simulink model "pHRIControl"  (Simulink 8.7)
settings: Solver=ode5  StartTime=0.0  StopTime=inf  FixedStep=0.01  RelTol=1e-3
InitFcn:
  | initpHRIControl
undefined symbols (not defined in the file or in its folder): CONFIG, HUMAN, ROBOT
libraries: WBToolboxLibrary x37
settings Model: Creator=yeshi  LastModifiedBy=yeshi  NumberOfSteps=50
settings DataIOCC: LimitDataPoints=off  SaveFormat=Dataset
settings DebuggingCC: UnderspecifiedInitializationDetection=Simplified  MergeDetectMultiDrivingBlocksExec=error
settings HardwareCC: ProdBitPerPointer=64  ProdLargestAtomicFloat=Float  ProdIntDivRoundTo=Zero  ProdEndianess=LittleEndian  ProdWordSize=64  ProdHWDeviceType=Intel->x86-64 (Windows64)
settings ModelReferenceCC: PropagateSignalLabelsOutOfModel=on
settings ConfigComp: CovModelRefEnable=off

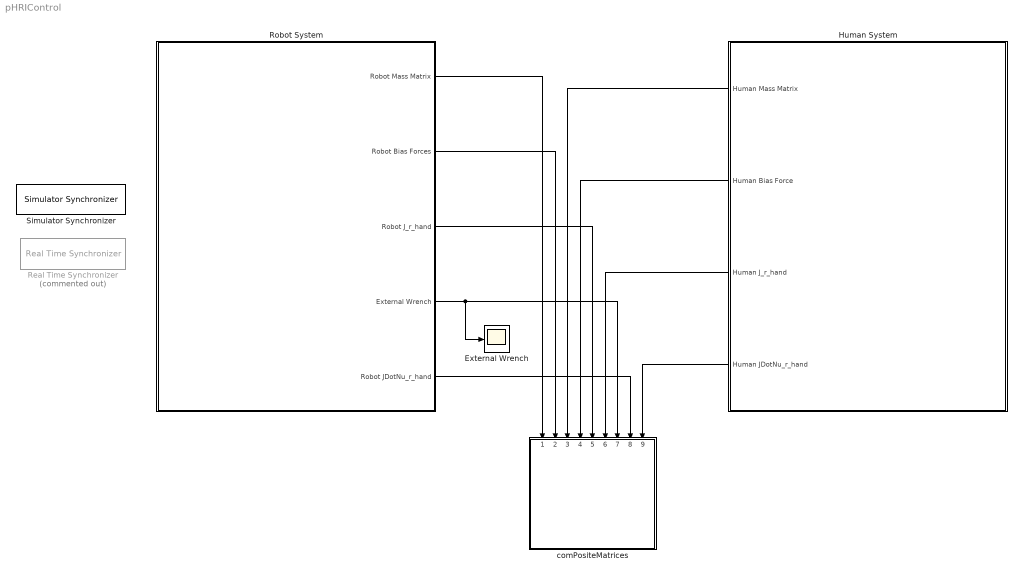
== system pHRIControl ==
  External Wrench : Scope
  Human System : Subsystem
  Real Time Synchronizer : WBToolboxLibrary/Utilities/Real Time Synchronizer  Commented=on  period=0.01
  Robot System : Subsystem
  Simulator Synchronizer : WBToolboxLibrary/Utilities/Simulator Synchronizer  period=0.01  serverPortName='/clock/rpc'  clientPortName='/WBT_synchronizer/rpc:o'
  comPositeMatrices : MATLAB Function  TreatAsAtomicUnit=on
  wires:
  Robot System/2(Robot Bias Forces) -> comPositeMatrices/2(robotBiasForce)
  Robot System/1(Robot Mass Matrix) -> comPositeMatrices/1(robotM)
  Human System/1(Human Mass Matrix) -> comPositeMatrices/3(humanM)
  Human System/2(Human Bias Force) -> comPositeMatrices/4(humanBiasForce)
  Robot System/3(Robot J_r_hand) -> comPositeMatrices/5(robotEEJ)
  Human System/3(Human J_r_hand) -> comPositeMatrices/6(humanEEJ)
  Robot System/5(Robot JDotNu_r_hand) -> comPositeMatrices/8(robotJDotNu)
  Human System/4(Human JDotNu_r_hand) -> comPositeMatrices/9(humanJDotNu)
  Robot System/4(External Wrench) -> External Wrench/1, comPositeMatrices/7(extWrench)

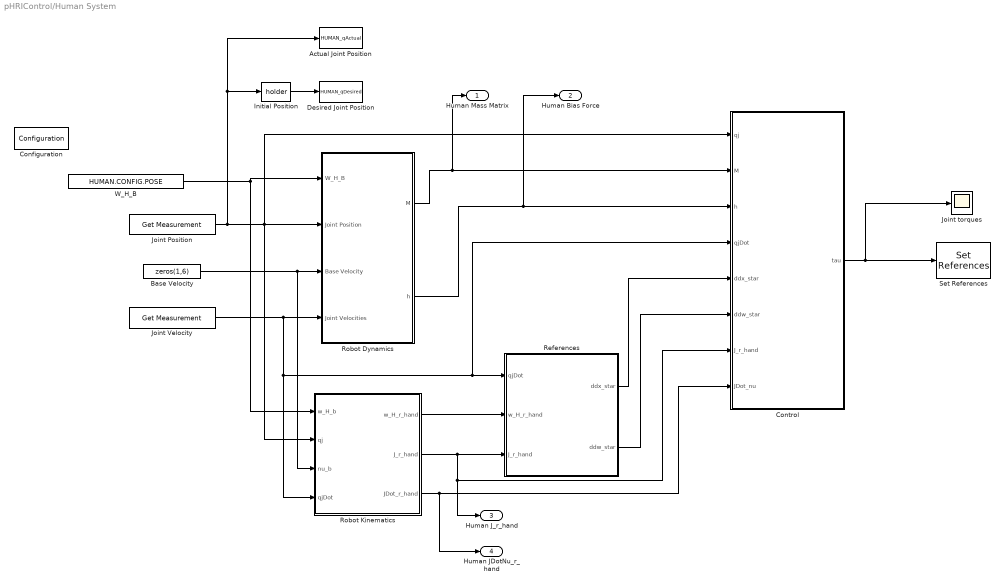
== system pHRIControl/Human System ==
  Actual Joint Position : ToWorkspace  VariableName=HUMAN_qActual  SaveFormat=Timeseries  SampleTime=-1
  "Base Velocity " : Constant  Value=zeros(1,6)
  Configuration : WBToolboxLibrary/Utilities/Configuration  ConfigSource=Workspace  ConfigObject='HUMAN.WBTConfigRobot'
  Control : Subsystem
  Desired Joint Position : ToWorkspace  VariableName=HUMAN_qDesired  SaveFormat=Timeseries  SampleTime=-1
  "Initial Position " : WBToolboxLibrary/Utilities/holder 
  Joint Position : WBToolboxLibrary/wholeBodyStates/Get Measurement  measuredType=Joints Position
  Joint Velocity : WBToolboxLibrary/wholeBodyStates/Get Measurement  measuredType=Joints Velocity
  Joint torques : Scope
  References : Subsystem
  Robot Dynamics : Subsystem
  Robot Kinematics : Subsystem
  Set References : WBToolboxLibrary/wholeBodyActuators/Set References  controlType=Torque  refSpeed=50
  "W_H_B " : Constant  Value=HUMAN.CONFIG.POSE
  Human Mass Matrix : Outport
  Human Bias Force : Outport  Port=2
  Human J_r_hand : Outport  Port=3
  Human JDotNu_r_hand : Outport  Port=4
  wires:
  Robot Dynamics/2(h) -> Human Bias Force/1, Control/3(h)
  "Base Velocity "/1 -> Robot Dynamics/3(Base Velocity), Robot Kinematics/3(nu_b)
  Robot Kinematics/2(J_r_hand) -> Human J_r_hand/1, Control/7(J_r_hand), References/3(J_r_hand)
  "Initial Position "/1 -> Desired Joint Position/1
  References/2(ddw_star) -> Control/6(ddw_star)
  References/1(ddx_star) -> Control/5(ddx_star)
  Control/1(tau) -> Joint torques/1, Set References/1
  Robot Kinematics/3(JDot_r_hand) -> Human JDotNu_r_hand/1, Control/8(JDot_nu)
  Robot Kinematics/1(w_H_r_hand) -> References/2(w_H_r_hand)
  Robot Dynamics/1(M) -> Human Mass Matrix/1, Control/2(M)
  "W_H_B "/1 -> Robot Dynamics/1(W_H_B), Robot Kinematics/1(w_H_b)
  Joint Velocity/1 -> Robot Dynamics/4(" Joint Velocities "), References/1(qjDot), Control/4(qjDot), Robot Kinematics/4(qjDot)
  Joint Position/1 -> "Initial Position "/1, Actual Joint Position/1, Robot Dynamics/2(Joint Position), Control/1(qj), Robot Kinematics/2(qj)

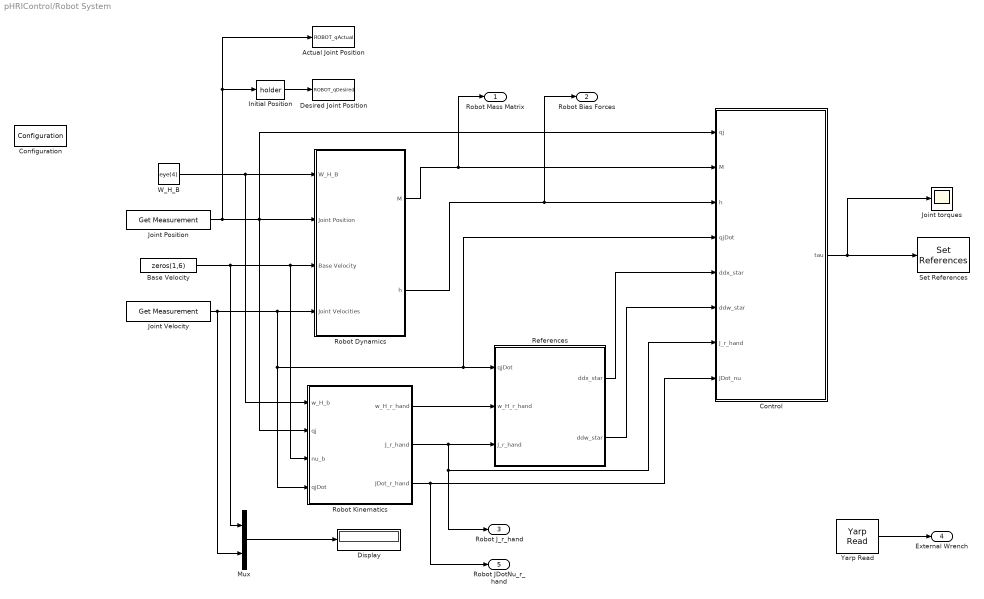
== system pHRIControl/Robot System ==
  Actual Joint Position : ToWorkspace  VariableName=ROBOT_qActual  SaveFormat=Timeseries  SampleTime=-1
  "Base Velocity " : Constant  Value=zeros(1,6)
  Configuration : WBToolboxLibrary/Utilities/Configuration  ConfigSource=Workspace  ConfigObject='ROBOT.WBTConfigRobot'
  Control : Subsystem
  Desired Joint Position : ToWorkspace  VariableName=ROBOT_qDesired  SaveFormat=Timeseries  SampleTime=-1
  Display : Display
  "Initial Position " : WBToolboxLibrary/Utilities/holder 
  Joint Position : WBToolboxLibrary/wholeBodyStates/Get Measurement  measuredType=Joints Position
  Joint Velocity : WBToolboxLibrary/wholeBodyStates/Get Measurement  measuredType=Joints Velocity
  Joint torques : Scope
  Mux : Mux  Inputs=2
  References : Subsystem
  Robot Dynamics : Subsystem
  Robot Kinematics : Subsystem
  Set References : WBToolboxLibrary/wholeBodyActuators/Set References  controlType=Torque  refSpeed=50
  "W_H_B " : Constant  Value=eye(4)
  Yarp Read : WBToolboxLibrary/Utilities/Yarp Read  portName='/iCub/wholeBodyDynamics/right_arm/endEffectorWrench:o'  signalSize=6  blocking=off  timestamp=off  autoconnect=on  errorOnConnection=on
  Robot Mass Matrix : Outport
  Robot Bias Forces : Outport  Port=2
  Robot J_r_hand : Outport  Port=3
  External Wrench : Outport  Port=4
  Robot JDotNu_r_hand : Outport  Port=5
  wires:
  Joint Position/1 -> Robot Kinematics/2(qj), Control/1(qj), Robot Dynamics/2(Joint Position), Actual Joint Position/1, "Initial Position "/1
  Joint Velocity/1 -> Mux/2, Robot Kinematics/4(qjDot), Control/4(qjDot), References/1(qjDot), Robot Dynamics/4(" Joint Velocities ")
  "W_H_B "/1 -> Robot Kinematics/1(w_H_b), Robot Dynamics/1(W_H_B)
  Robot Dynamics/1(M) -> Control/2(M), Robot Mass Matrix/1
  Robot Kinematics/1(w_H_r_hand) -> References/2(w_H_r_hand)
  Robot Kinematics/3(JDot_r_hand) -> Robot JDotNu_r_hand/1, Control/8(JDot_nu)
  Control/1(tau) -> Set References/1, Joint torques/1
  References/1(ddx_star) -> Control/5(ddx_star)
  References/2(ddw_star) -> Control/6(ddw_star)
  "Initial Position "/1 -> Desired Joint Position/1
  Robot Kinematics/2(J_r_hand) -> References/3(J_r_hand), Robot J_r_hand/1, Control/7(J_r_hand)
  "Base Velocity "/1 -> Mux/1, Robot Kinematics/3(nu_b), Robot Dynamics/3(Base Velocity)
  Robot Dynamics/2(h) -> Robot Bias Forces/1, Control/3(h)
  Yarp Read/1 -> External Wrench/1
  Mux/1 -> Display/1

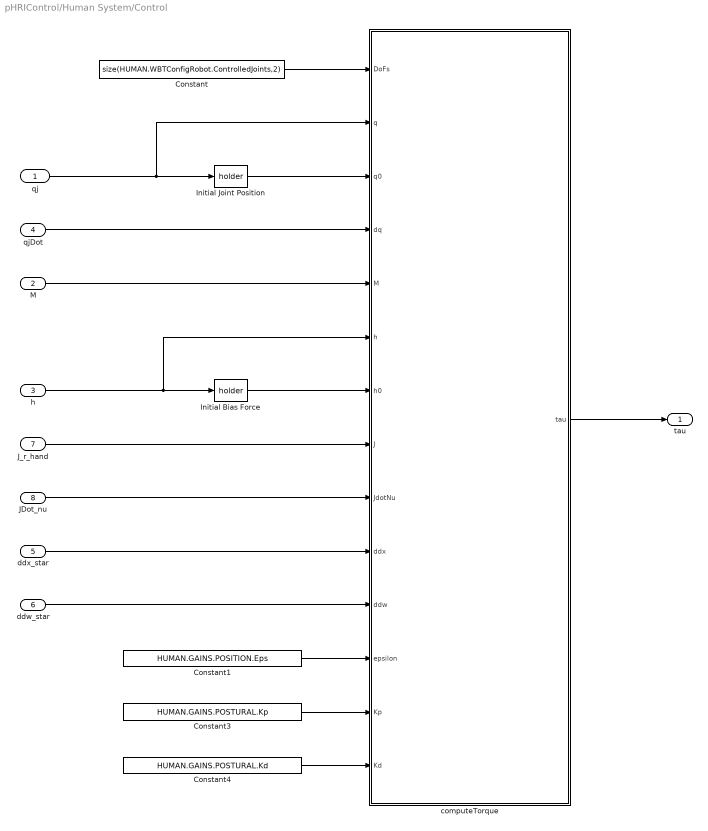
== system pHRIControl/Human System/Control ==
  qj : Inport
  M : Inport  Port=2
  h : Inport  Port=3
  qjDot : Inport  Port=4
  ddx_star : Inport  Port=5
  ddw_star : Inport  Port=6
  J_r_hand : Inport  Port=7
  JDot_nu : Inport  Port=8
  Constant : Constant  Value=size(HUMAN.WBTConfigRobot.ControlledJoints,2)
  Constant1 : Constant  Value=HUMAN.GAINS.POSITION.Eps
  Constant3 : Constant  Value=HUMAN.GAINS.POSTURAL.Kp
  Constant4 : Constant  Value=HUMAN.GAINS.POSTURAL.Kd
  Initial Bias Force : WBToolboxLibrary/Utilities/holder 
  Initial Joint Position : WBToolboxLibrary/Utilities/holder 
  computeTorque : MATLAB Function  TreatAsAtomicUnit=on
  tau : Outport
  wires:
  Constant4/1 -> computeTorque/14(Kd)
  Constant3/1 -> computeTorque/13(Kp)
  Constant1/1 -> computeTorque/12(epsilon)
  ddw_star/1 -> computeTorque/11(ddw)
  M/1 -> computeTorque/5(M)
  J_r_hand/1 -> computeTorque/8(J)
  Initial Joint Position/1 -> computeTorque/3(q0)
  Initial Bias Force/1 -> computeTorque/7(h0)
  h/1 -> Initial Bias Force/1, computeTorque/6(h)
  computeTorque/1(tau) -> tau/1
  Constant/1 -> computeTorque/1(DoFs)
  JDot_nu/1 -> computeTorque/9(JdotNu)
  qjDot/1 -> computeTorque/4(dq)
  qj/1 -> Initial Joint Position/1, computeTorque/2(q)
  ddx_star/1 -> computeTorque/10(ddx)

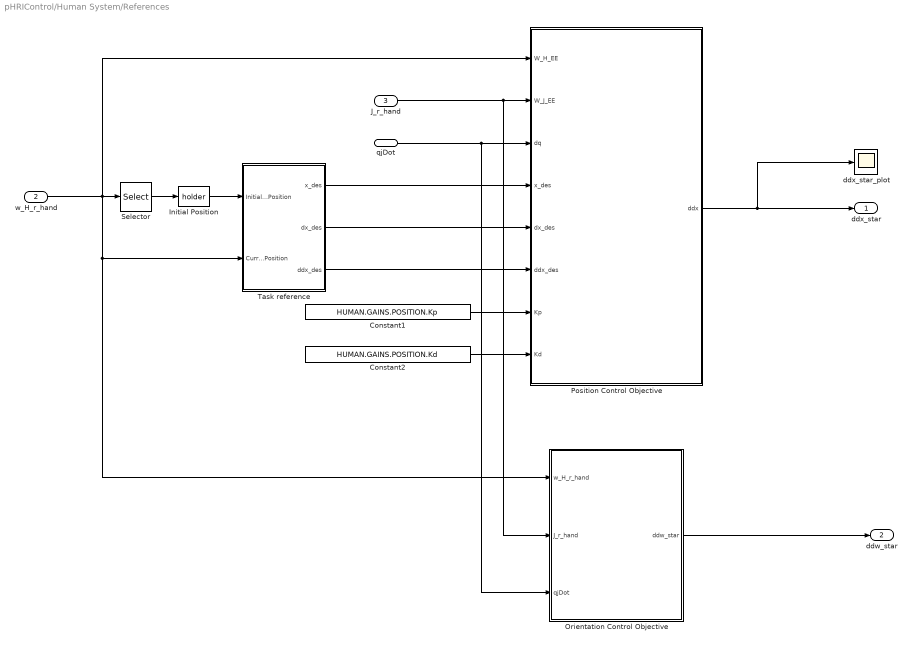
== system pHRIControl/Human System/References ==
  qjDot : Inport
  w_H_r_hand : Inport  Port=2
  J_r_hand : Inport  Port=3
  Constant1 : Constant  Value=HUMAN.GAINS.POSITION.Kp
  Constant2 : Constant  Value=HUMAN.GAINS.POSITION.Kd
  "Initial Position " : WBToolboxLibrary/Utilities/holder 
  Orientation Control Objective : Subsystem
  Position Control Objective : MATLAB Function  TreatAsAtomicUnit=on
  Selector : Selector  NumberOfDimensions=2  InputPortWidth=3  IndexOptions=Index vector (dialog),Index vector (dialog)  Indices=[1 2 3],4  OutputSizes=1,1
  Task reference : Subsystem
  ddx_star_plot : Scope
  ddx_star : Outport
  ddw_star : Outport  Port=2
  wires:
  Orientation Control Objective/1(ddw_star) -> ddw_star/1
  Constant2/1 -> Position Control Objective/8(Kd)
  Constant1/1 -> Position Control Objective/7(Kp)
  w_H_r_hand/1 -> Task reference/2(Current Position), Orientation Control Objective/1(w_H_r_hand), Position Control Objective/1(W_H_EE), Selector/1
  qjDot/1 -> Position Control Objective/3(dq), Orientation Control Objective/3(qjDot)
  Selector/1 -> "Initial Position "/1
  Position Control Objective/1(ddx) -> ddx_star_plot/1, ddx_star/1
  "Initial Position "/1 -> Task reference/1(Initial Position)
  Task reference/3(ddx_des) -> Position Control Objective/6(ddx_des)
  Task reference/2(dx_des) -> Position Control Objective/5(dx_des)
  Task reference/1(x_des) -> Position Control Objective/4(x_des)
  J_r_hand/1 -> Position Control Objective/2(W_J_EE), Orientation Control Objective/2(J_r_hand)

== system pHRIControl/Human System/Robot Dynamics ==
  W_H_B : Inport
  Joint Position : Inport  Port=2
  Base Velocity : Inport  Port=3
  " Joint Velocities " : Inport  Port=4
  Get Bias Forces : WBToolboxLibrary/wholeBodyModel/Dynamics/Get Bias Forces
  Mass Matrix : WBToolboxLibrary/wholeBodyModel/Dynamics/Mass Matrix
  M : Outport
  h : Outport  Port=2
  wires:
  Mass Matrix/1 -> M/1
  Base Velocity/1 -> Get Bias Forces/3
  W_H_B/1 -> Get Bias Forces/1, Mass Matrix/1
  Get Bias Forces/1 -> h/1
  " Joint Velocities "/1 -> Get Bias Forces/4
  Joint Position/1 -> Get Bias Forces/2, Mass Matrix/2

== system pHRIControl/Human System/Robot Kinematics ==
  w_H_b : Inport
  qj : Inport  Port=2
  nu_b : Inport  Port=3
  qjDot : Inport  Port=4
  DotJ Nu : WBToolboxLibrary/wholeBodyModel/Jacobians/DotJ Nu  frameName=HUMAN.CONFIG.EE
  Forward Kinematics : WBToolboxLibrary/wholeBodyModel/Kinematics/Forward Kinematics  frameName=HUMAN.CONFIG.EE
  Jacobian 6x(6+n) : WBToolboxLibrary/wholeBodyModel/Jacobians/Jacobian  frameName=HUMAN.CONFIG.EE
  w_H_r_hand : Outport
  J_r_hand : Outport  Port=2
  JDot_r_hand : Outport  Port=3
  wires:
  DotJ Nu/1 -> JDot_r_hand/1
  Forward Kinematics/1 -> w_H_r_hand/1
  Jacobian 6x(6+n)/1 -> J_r_hand/1
  nu_b/1 -> DotJ Nu/3
  qjDot/1 -> DotJ Nu/4
  qj/1 -> Forward Kinematics/2, Jacobian 6x(6+n)/2, DotJ Nu/2
  w_H_b/1 -> Forward Kinematics/1, Jacobian 6x(6+n)/1, DotJ Nu/1

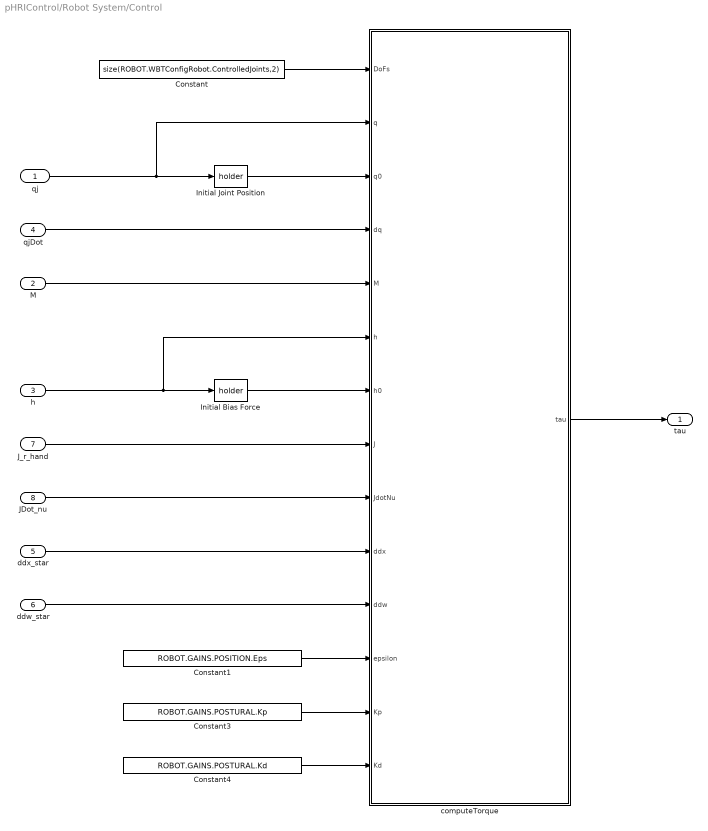
== system pHRIControl/Robot System/Control ==
  qj : Inport
  M : Inport  Port=2
  h : Inport  Port=3
  qjDot : Inport  Port=4
  ddx_star : Inport  Port=5
  ddw_star : Inport  Port=6
  J_r_hand : Inport  Port=7
  JDot_nu : Inport  Port=8
  Constant : Constant  Value=size(ROBOT.WBTConfigRobot.ControlledJoints,2)
  Constant1 : Constant  Value=ROBOT.GAINS.POSITION.Eps
  Constant3 : Constant  Value=ROBOT.GAINS.POSTURAL.Kp
  Constant4 : Constant  Value=ROBOT.GAINS.POSTURAL.Kd
  Initial Bias Force : WBToolboxLibrary/Utilities/holder 
  Initial Joint Position : WBToolboxLibrary/Utilities/holder 
  computeTorque : MATLAB Function  TreatAsAtomicUnit=on
  tau : Outport
  wires:
  ddx_star/1 -> computeTorque/10(ddx)
  qj/1 -> computeTorque/2(q), Initial Joint Position/1
  qjDot/1 -> computeTorque/4(dq)
  JDot_nu/1 -> computeTorque/9(JdotNu)
  Constant/1 -> computeTorque/1(DoFs)
  computeTorque/1(tau) -> tau/1
  h/1 -> computeTorque/6(h), Initial Bias Force/1
  Initial Bias Force/1 -> computeTorque/7(h0)
  Initial Joint Position/1 -> computeTorque/3(q0)
  J_r_hand/1 -> computeTorque/8(J)
  M/1 -> computeTorque/5(M)
  ddw_star/1 -> computeTorque/11(ddw)
  Constant1/1 -> computeTorque/12(epsilon)
  Constant3/1 -> computeTorque/13(Kp)
  Constant4/1 -> computeTorque/14(Kd)

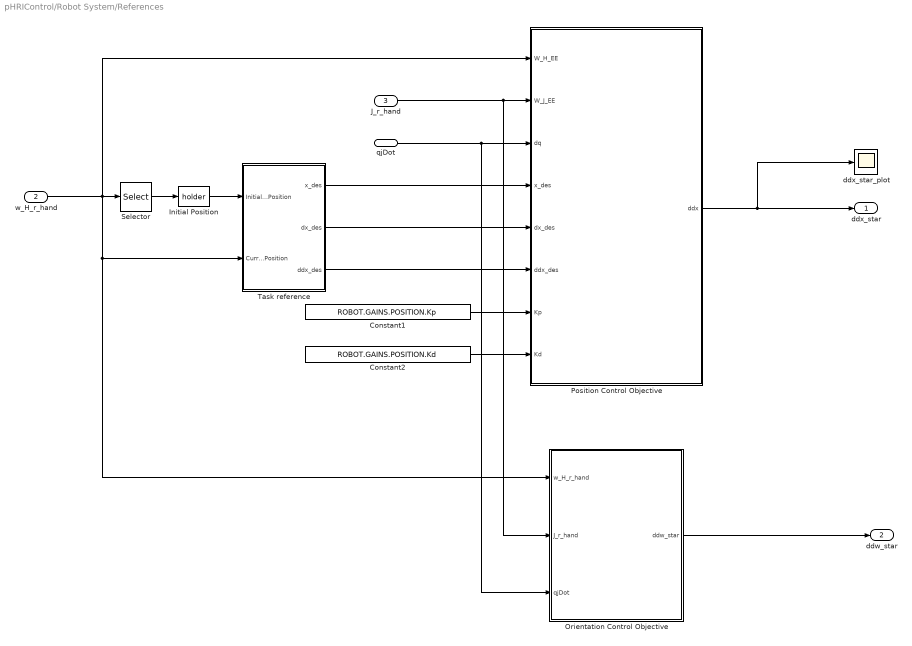
== system pHRIControl/Robot System/References ==
  qjDot : Inport
  w_H_r_hand : Inport  Port=2
  J_r_hand : Inport  Port=3
  Constant1 : Constant  Value=ROBOT.GAINS.POSITION.Kp
  Constant2 : Constant  Value=ROBOT.GAINS.POSITION.Kd
  "Initial Position " : WBToolboxLibrary/Utilities/holder 
  Orientation Control Objective : Subsystem
  Position Control Objective : MATLAB Function  TreatAsAtomicUnit=on
  Selector : Selector  NumberOfDimensions=2  InputPortWidth=3  IndexOptions=Index vector (dialog),Index vector (dialog)  Indices=[1 2 3],4  OutputSizes=1,1
  Task reference : Subsystem
  ddx_star_plot : Scope
  ddx_star : Outport
  ddw_star : Outport  Port=2
  wires:
  J_r_hand/1 -> Orientation Control Objective/2(J_r_hand), Position Control Objective/2(W_J_EE)
  Task reference/1(x_des) -> Position Control Objective/4(x_des)
  Task reference/2(dx_des) -> Position Control Objective/5(dx_des)
  Task reference/3(ddx_des) -> Position Control Objective/6(ddx_des)
  "Initial Position "/1 -> Task reference/1(Initial Position)
  Position Control Objective/1(ddx) -> ddx_star/1, ddx_star_plot/1
  Selector/1 -> "Initial Position "/1
  qjDot/1 -> Orientation Control Objective/3(qjDot), Position Control Objective/3(dq)
  w_H_r_hand/1 -> Selector/1, Position Control Objective/1(W_H_EE), Orientation Control Objective/1(w_H_r_hand), Task reference/2(Current Position)
  Constant1/1 -> Position Control Objective/7(Kp)
  Constant2/1 -> Position Control Objective/8(Kd)
  Orientation Control Objective/1(ddw_star) -> ddw_star/1

== system pHRIControl/Robot System/Robot Dynamics ==
  W_H_B : Inport
  Joint Position : Inport  Port=2
  Base Velocity : Inport  Port=3
  " Joint Velocities " : Inport  Port=4
  Get Bias Forces : WBToolboxLibrary/wholeBodyModel/Dynamics/Get Bias Forces
  Mass Matrix : WBToolboxLibrary/wholeBodyModel/Dynamics/Mass Matrix
  M : Outport
  h : Outport  Port=2
  wires:
  Joint Position/1 -> Mass Matrix/2, Get Bias Forces/2
  " Joint Velocities "/1 -> Get Bias Forces/4
  Get Bias Forces/1 -> h/1
  W_H_B/1 -> Mass Matrix/1, Get Bias Forces/1
  Base Velocity/1 -> Get Bias Forces/3
  Mass Matrix/1 -> M/1

== system pHRIControl/Robot System/Robot Kinematics ==
  w_H_b : Inport
  qj : Inport  Port=2
  nu_b : Inport  Port=3
  qjDot : Inport  Port=4
  DotJ Nu : WBToolboxLibrary/wholeBodyModel/Jacobians/DotJ Nu  frameName=ROBOT.CONFIG.EE
  Forward Kinematics : WBToolboxLibrary/wholeBodyModel/Kinematics/Forward Kinematics  frameName=ROBOT.CONFIG.EE
  Jacobian 6x(6+n) : WBToolboxLibrary/wholeBodyModel/Jacobians/Jacobian  frameName=ROBOT.CONFIG.EE
  w_H_r_hand : Outport
  J_r_hand : Outport  Port=2
  JDot_r_hand : Outport  Port=3
  wires:
  w_H_b/1 -> DotJ Nu/1, Jacobian 6x(6+n)/1, Forward Kinematics/1
  qj/1 -> DotJ Nu/2, Jacobian 6x(6+n)/2, Forward Kinematics/2
  qjDot/1 -> DotJ Nu/4
  nu_b/1 -> DotJ Nu/3
  Jacobian 6x(6+n)/1 -> J_r_hand/1
  Forward Kinematics/1 -> w_H_r_hand/1
  DotJ Nu/1 -> JDot_r_hand/1

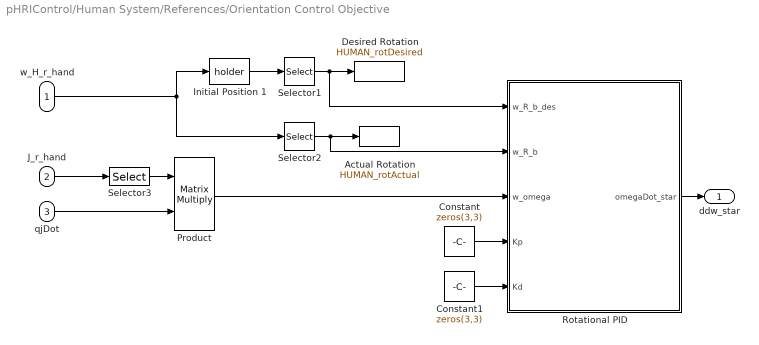
== system pHRIControl/Human System/References/Orientation Control Objective ==
  w_H_r_hand : Inport
  J_r_hand : Inport  Port=2
  qjDot : Inport  Port=3
  Actual Rotation : ToWorkspace  VariableName=HUMAN_rotActual  SaveFormat=Timeseries  SampleTime=-1
  Constant : Constant  Value=zeros(3,3)
  Constant1 : Constant  Value=zeros(3,3)
  Desired Rotation : ToWorkspace  VariableName=HUMAN_rotDesired  SaveFormat=Timeseries  SampleTime=-1
  Initial Position 1 : WBToolboxLibrary/Utilities/holder 
  Product : Product  Multiplication=Matrix(*)
  Rotational PID : MATLAB Function  TreatAsAtomicUnit=on
  Selector1 : Selector  NumberOfDimensions=2  InputPortWidth=4  IndexOptions=Index vector (dialog),Index vector (dialog)  Indices=[1:3],[1:3]  OutputSizes=1,1
  Selector2 : Selector  NumberOfDimensions=2  InputPortWidth=4  IndexOptions=Index vector (dialog),Index vector (dialog)  Indices=[1:3],[1:3]  OutputSizes=1,1
  Selector3 : Selector  NumberOfDimensions=2  InputPortWidth=4  IndexOptions=Index vector (dialog),Index vector (dialog)  Indices=[4:6],[7:6+11]  OutputSizes=1,1
  ddw_star : Outport
  wires:
  Product/1 -> Rotational PID/3(w_omega)
  qjDot/1 -> Product/2
  Selector3/1 -> Product/1
  J_r_hand/1 -> Selector3/1
  Constant1/1 -> Rotational PID/5(Kd)
  Constant/1 -> Rotational PID/4(Kp)
  Initial Position 1/1 -> Selector1/1
  w_H_r_hand/1 -> Initial Position 1/1, Selector2/1
  Selector1/1 -> Rotational PID/1(w_R_b_des), Desired Rotation/1
  Rotational PID/1(omegaDot_star) -> ddw_star/1
  Selector2/1 -> Actual Rotation/1, Rotational PID/2(w_R_b)

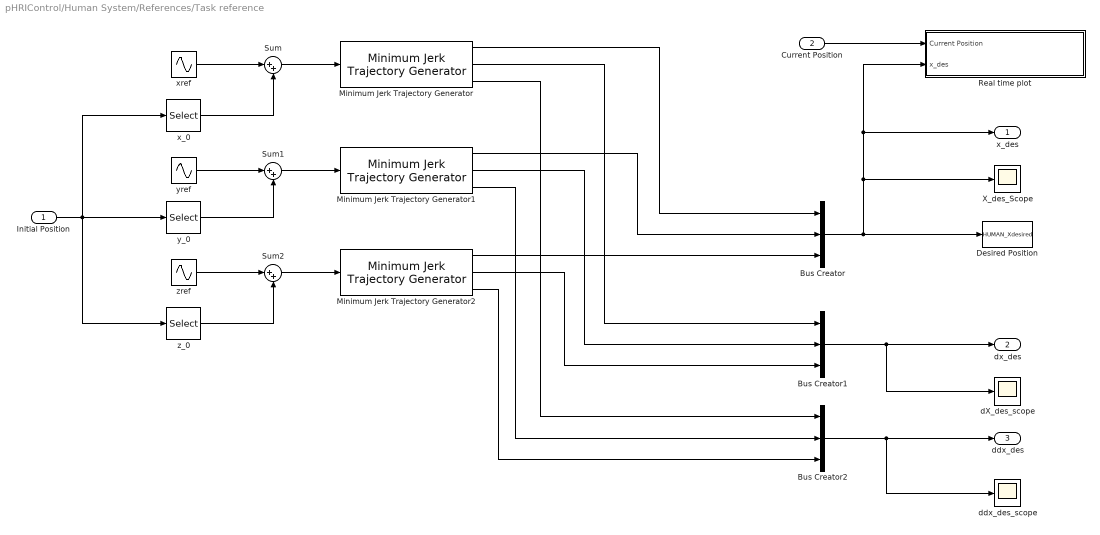
== system pHRIControl/Human System/References/Task reference ==
  Initial Position : Inport
  Current Position : Inport  Port=2
  Bus Creator : BusCreator  Inputs=3
  Bus Creator1 : BusCreator  Inputs=3
  Bus Creator2 : BusCreator  Inputs=3
  Desired Position : ToWorkspace  VariableName=HUMAN_Xdesired  SaveFormat=Timeseries  SampleTime=-1
  Minimum Jerk Trajectory Generator : WBToolboxLibrary/Utilities/Minimum Jerk Trajectory Generator  externalSettlingTime=off  settlingTime=3  sampleTime=0.01  resetOnSettlingTime=off  firstDerivatives=on  secondDerivatives=on  explicitInitialValue=off
  Minimum Jerk Trajectory Generator1 : WBToolboxLibrary/Utilities/Minimum Jerk Trajectory Generator  externalSettlingTime=off  settlingTime=3  sampleTime=0.01  resetOnSettlingTime=off  firstDerivatives=on  secondDerivatives=on  explicitInitialValue=off
  Minimum Jerk Trajectory Generator2 : WBToolboxLibrary/Utilities/Minimum Jerk Trajectory Generator  externalSettlingTime=off  settlingTime=3  sampleTime=0.01  resetOnSettlingTime=off  firstDerivatives=on  secondDerivatives=on  explicitInitialValue=off
  Real time plot : Subsystem
  Sum : Sum  Inputs=|++
  Sum1 : Sum  Inputs=|++
  Sum2 : Sum  Inputs=|++
  X_des_Scope : Scope
  dX_des_scope : Scope
  ddx_des_scope : Scope
  x_0 : Selector  InputPortWidth=3  IndexOptions=Index vector (dialog)  Indices=[1]  OutputSizes=1
  xref : Sin  Amplitude=0  SampleTime=0
  y_0 : Selector  InputPortWidth=3  IndexOptions=Index vector (dialog)  Indices=[2]  OutputSizes=1
  yref : Sin  Amplitude=0  SampleTime=0
  z_0 : Selector  InputPortWidth=3  IndexOptions=Index vector (dialog)  Indices=[3]  OutputSizes=1
  zref : Sin  Amplitude=0  Phase=pi/2  SampleTime=0
  x_des : Outport
  dx_des : Outport  Port=2
  ddx_des : Outport  Port=3
  wires:
  Current Position/1 -> Real time plot/1(Current Position)
  x_0/1 -> Sum/2
  Initial Position/1 -> z_0/1, y_0/1, x_0/1
  z_0/1 -> Sum2/2
  Sum/1 -> Minimum Jerk Trajectory Generator/1
  Minimum Jerk Trajectory Generator/2 -> Bus Creator1/1
  xref/1 -> Sum/1
  Minimum Jerk Trajectory Generator1/1 -> Bus Creator/2
  Bus Creator/1 -> X_des_Scope/1, x_des/1, Real time plot/2(x_des), Desired Position/1
  Bus Creator2/1 -> ddx_des_scope/1, ddx_des/1
  Minimum Jerk Trajectory Generator1/2 -> Bus Creator1/2
  zref/1 -> Sum2/1
  Bus Creator1/1 -> dX_des_scope/1, dx_des/1
  Minimum Jerk Trajectory Generator2/3 -> Bus Creator2/3
  Sum1/1 -> Minimum Jerk Trajectory Generator1/1
  y_0/1 -> Sum1/2
  Minimum Jerk Trajectory Generator1/3 -> Bus Creator2/2
  Minimum Jerk Trajectory Generator/1 -> Bus Creator/1
  yref/1 -> Sum1/1
  Minimum Jerk Trajectory Generator/3 -> Bus Creator2/1
  Minimum Jerk Trajectory Generator2/1 -> Bus Creator/3
  Sum2/1 -> Minimum Jerk Trajectory Generator2/1
  Minimum Jerk Trajectory Generator2/2 -> Bus Creator1/3

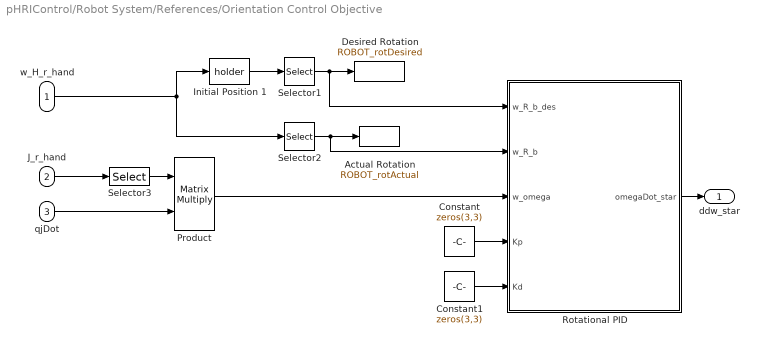
== system pHRIControl/Robot System/References/Orientation Control Objective ==
  w_H_r_hand : Inport
  J_r_hand : Inport  Port=2
  qjDot : Inport  Port=3
  Actual Rotation : ToWorkspace  VariableName=ROBOT_rotActual  SaveFormat=Timeseries  SampleTime=-1
  Constant : Constant  Value=zeros(3,3)
  Constant1 : Constant  Value=zeros(3,3)
  Desired Rotation : ToWorkspace  VariableName=ROBOT_rotDesired  SaveFormat=Timeseries  SampleTime=-1
  Initial Position 1 : WBToolboxLibrary/Utilities/holder 
  Product : Product  Multiplication=Matrix(*)
  Rotational PID : MATLAB Function  TreatAsAtomicUnit=on
  Selector1 : Selector  NumberOfDimensions=2  InputPortWidth=4  IndexOptions=Index vector (dialog),Index vector (dialog)  Indices=[1:3],[1:3]  OutputSizes=1,1
  Selector2 : Selector  NumberOfDimensions=2  InputPortWidth=4  IndexOptions=Index vector (dialog),Index vector (dialog)  Indices=[1:3],[1:3]  OutputSizes=1,1
  Selector3 : Selector  NumberOfDimensions=2  InputPortWidth=4  IndexOptions=Index vector (dialog),Index vector (dialog)  Indices=[4:6],[7:6+11]  OutputSizes=1,1
  ddw_star : Outport
  wires:
  Selector2/1 -> Rotational PID/2(w_R_b), Actual Rotation/1
  Rotational PID/1(omegaDot_star) -> ddw_star/1
  Selector1/1 -> Desired Rotation/1, Rotational PID/1(w_R_b_des)
  w_H_r_hand/1 -> Selector2/1, Initial Position 1/1
  Initial Position 1/1 -> Selector1/1
  Constant/1 -> Rotational PID/4(Kp)
  Constant1/1 -> Rotational PID/5(Kd)
  J_r_hand/1 -> Selector3/1
  Selector3/1 -> Product/1
  qjDot/1 -> Product/2
  Product/1 -> Rotational PID/3(w_omega)

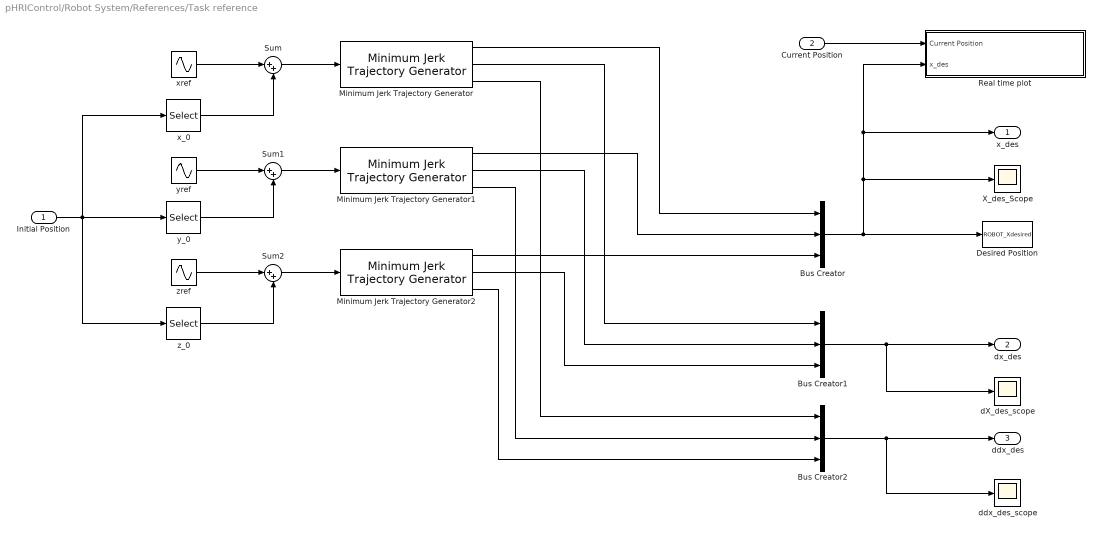
== system pHRIControl/Robot System/References/Task reference ==
  Initial Position : Inport
  Current Position : Inport  Port=2
  Bus Creator : BusCreator  Inputs=3
  Bus Creator1 : BusCreator  Inputs=3
  Bus Creator2 : BusCreator  Inputs=3
  Desired Position : ToWorkspace  VariableName=ROBOT_Xdesired  SaveFormat=Timeseries  SampleTime=-1
  Minimum Jerk Trajectory Generator : WBToolboxLibrary/Utilities/Minimum Jerk Trajectory Generator  externalSettlingTime=off  settlingTime=3  sampleTime=0.01  resetOnSettlingTime=off  firstDerivatives=on  secondDerivatives=on  explicitInitialValue=off
  Minimum Jerk Trajectory Generator1 : WBToolboxLibrary/Utilities/Minimum Jerk Trajectory Generator  externalSettlingTime=off  settlingTime=3  sampleTime=0.01  resetOnSettlingTime=off  firstDerivatives=on  secondDerivatives=on  explicitInitialValue=off
  Minimum Jerk Trajectory Generator2 : WBToolboxLibrary/Utilities/Minimum Jerk Trajectory Generator  externalSettlingTime=off  settlingTime=3  sampleTime=0.01  resetOnSettlingTime=off  firstDerivatives=on  secondDerivatives=on  explicitInitialValue=off
  Real time plot : Subsystem
  Sum : Sum  Inputs=|++
  Sum1 : Sum  Inputs=|++
  Sum2 : Sum  Inputs=|++
  X_des_Scope : Scope
  dX_des_scope : Scope
  ddx_des_scope : Scope
  x_0 : Selector  InputPortWidth=3  IndexOptions=Index vector (dialog)  Indices=[1]  OutputSizes=1
  xref : Sin  Amplitude=0  SampleTime=0
  y_0 : Selector  InputPortWidth=3  IndexOptions=Index vector (dialog)  Indices=[2]  OutputSizes=1
  yref : Sin  Amplitude=0.15  SampleTime=0
  z_0 : Selector  InputPortWidth=3  IndexOptions=Index vector (dialog)  Indices=[3]  OutputSizes=1
  zref : Sin  Amplitude=0  Phase=pi/2  SampleTime=0
  x_des : Outport
  dx_des : Outport  Port=2
  ddx_des : Outport  Port=3
  wires:
  Minimum Jerk Trajectory Generator2/2 -> Bus Creator1/3
  Sum2/1 -> Minimum Jerk Trajectory Generator2/1
  Minimum Jerk Trajectory Generator2/1 -> Bus Creator/3
  Minimum Jerk Trajectory Generator/3 -> Bus Creator2/1
  yref/1 -> Sum1/1
  Minimum Jerk Trajectory Generator/1 -> Bus Creator/1
  Minimum Jerk Trajectory Generator1/3 -> Bus Creator2/2
  y_0/1 -> Sum1/2
  Sum1/1 -> Minimum Jerk Trajectory Generator1/1
  Minimum Jerk Trajectory Generator2/3 -> Bus Creator2/3
  Bus Creator1/1 -> dx_des/1, dX_des_scope/1
  zref/1 -> Sum2/1
  Minimum Jerk Trajectory Generator1/2 -> Bus Creator1/2
  Bus Creator2/1 -> ddx_des/1, ddx_des_scope/1
  Bus Creator/1 -> Desired Position/1, Real time plot/2(x_des), x_des/1, X_des_Scope/1
  Minimum Jerk Trajectory Generator1/1 -> Bus Creator/2
  xref/1 -> Sum/1
  Minimum Jerk Trajectory Generator/2 -> Bus Creator1/1
  Sum/1 -> Minimum Jerk Trajectory Generator/1
  z_0/1 -> Sum2/2
  Initial Position/1 -> x_0/1, y_0/1, z_0/1
  x_0/1 -> Sum/2
  Current Position/1 -> Real time plot/1(Current Position)

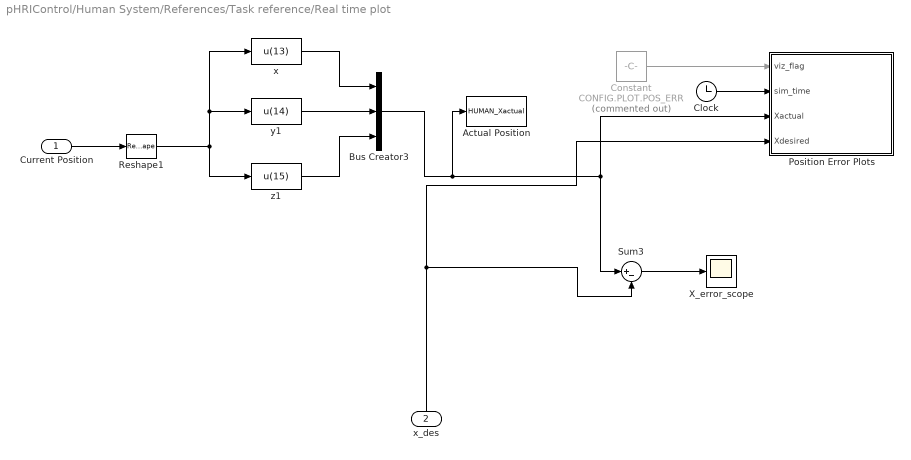
== system pHRIControl/Human System/References/Task reference/Real time plot ==
  Current Position : Inport
  x_des : Inport  Port=2
  Actual Position : ToWorkspace  VariableName=HUMAN_Xactual  SaveFormat=Timeseries  SampleTime=-1
  Bus Creator3 : BusCreator  Inputs=3
  Clock : Clock
  Constant : Constant  Commented=on  Value=CONFIG.PLOT.POS_ERR
  "Position Error Plots " : MATLAB Function  TreatAsAtomicUnit=on
  Reshape1 : Reshape
  Sum3 : Sum  Inputs=|+-
  X_error_scope : Scope
  x : Fcn  Expr=u(13)
  y1 : Fcn  Expr=u(14)
  z1 : Fcn  Expr=u(15)
  wires:
  Sum3/1 -> X_error_scope/1
  Constant/1 -> "Position Error Plots "/1(viz_flag)
  Bus Creator3/1 -> "Position Error Plots "/3(Xactual), Sum3/1, Actual Position/1
  Clock/1 -> "Position Error Plots "/2(sim_time)
  z1/1 -> Bus Creator3/3
  y1/1 -> Bus Creator3/2
  x/1 -> Bus Creator3/1
  Reshape1/1 -> z1/1, y1/1, x/1
  Current Position/1 -> Reshape1/1
  x_des/1 -> "Position Error Plots "/4(Xdesired), Sum3/2

== system pHRIControl/Robot System/References/Task reference/Real time plot ==
  Current Position : Inport
  x_des : Inport  Port=2
  Actual Position : ToWorkspace  VariableName=ROBOT_Xactual  SaveFormat=Timeseries  SampleTime=-1
  Bus Creator3 : BusCreator  Inputs=3
  Clock : Clock
  Constant : Constant  Commented=on  Value=CONFIG.PLOT.POS_ERR
  "Position Error Plots " : MATLAB Function  TreatAsAtomicUnit=on
  Reshape1 : Reshape
  Sum3 : Sum  Inputs=|+-
  X_error_scope : Scope
  x : Fcn  Expr=u(13)
  y1 : Fcn  Expr=u(14)
  z1 : Fcn  Expr=u(15)
  wires:
  x_des/1 -> Sum3/2, "Position Error Plots "/4(Xdesired)
  Current Position/1 -> Reshape1/1
  Reshape1/1 -> x/1, y1/1, z1/1
  x/1 -> Bus Creator3/1
  y1/1 -> Bus Creator3/2
  z1/1 -> Bus Creator3/3
  Clock/1 -> "Position Error Plots "/2(sim_time)
  Bus Creator3/1 -> Actual Position/1, Sum3/1, "Position Error Plots "/3(Xactual)
  Constant/1 -> "Position Error Plots "/1(viz_flag)
  Sum3/1 -> X_error_scope/1

== matlab function Robot System/References/Position Control Objective ==
  data: W_H_EE input double; ddx output double; W_J_EE input double; dq input double; x_des input double; dx_des input double; ddx_des input double; Kp input double; Kd input double
function ddx = controlObjective(W_H_EE,W_J_EE,dq,x_des,dx_des,ddx_des,Kp,Kd)
   
    x  = W_H_EE(1:3,4)-x_des;
    dx = W_J_EE(1:3,7:end)*dq-dx_des;
    
    ddx = ddx_des-Kp*x-Kd*dx; 

end

== matlab function Robot System/Control/computeTorque ==
  data: DoFs input double; q input double; q0 input double; dq input double; M input double; h input double; h0 input double; J input double; JdotNu input double; ddx input double; tau output double; ddw input double; epsilon input double; Kp input double; Kd input double
function tau   = computeTorque(DoFs,q,q0,dq,M,h,h0,J,JdotNu,ddx,ddw,epsilon,Kp,Kd)

    Dofs = 11;
    
    Sb = zeros(Dofs,6);
    Ss = eye(Dofs);
    S = [Sb Ss]';

    ddX = [ddx' 0 0 0]';

    %%Primary Task
    lambda = (J(1:3,:)/M)*S;
    alpha = pinvDamped(lambda,epsilon);
    
    tau_pri = alpha*(ddX(1:3) - JdotNu(1:3) + (J(1:3,:)/M)*h);
    
    nullspace = eye(size(lambda,2)) - alpha*lambda;
    
    %%Postural Task
    kp = Kp;
    kd = Kd;
    tau_null = S'*h - kp*(q-q0) - kd*(dq);
    
    tau = tau_pri + nullspace*tau_null;

end

== matlab function Robot System/References/Task reference/Real time plot/Position Error Plots  ==
  data: viz_flag input double; sim_time input double; Xactual input double; Xdesired input double
function positionErrorPlots(viz_flag,sim_time,Xactual,Xdesired)
%#codegen

coder.extrinsic('animatedline')
coder.extrinsic('addpoints')
coder.extrinsic('legend')
coder.extrinsic('clearpoints')

if(viz_flag ~= 0)
    
    Xerror = Xactual - Xdesired;
    curve_position_error = animatedline('LineWidth',0.1,'Marker','+');

    if(sim_time == 0)
    
        clf;
        close;
    
        fig1 = figure;
        view(177,15); hold on;
        grid on;
        xlabel('x');
        ylabel('y');
        zlabel('z');
        title('Position Error'); hold on;
% %         axis([-0.3 0.3 -0.3 0.3 -0.3 0.3]);
       
    end
    
    figure(1);
    addpoints(curve_position_error,Xerror(1),Xerror(2),Xerror(3));
    drawnow;
    
end

end

== matlab function Robot System/References/Orientation Control Objective/Rotational PID ==
  data: w_R_b_des input double; w_R_b input double; w_omega input double; omegaDot_star output double; Kp input double; Kd input double
function omegaDot_star = rotPID(w_R_b_des,w_R_b,w_omega,Kp,Kd)

    w_omega_des = [0;0;0];
    w_omegaDot_des = [0;0;0];
    
    omegaDot_star = rotationalPID(w_R_b,w_omega,w_R_b_des,w_omega_des,w_omegaDot_des,Kp,Kd);
end

== matlab function Human System/Control/computeTorque ==
  data: DoFs input double; q input double; q0 input double; dq input double; M input double; h input double; h0 input double; J input double; JdotNu input double; ddx input double; tau output double; ddw input double; epsilon input double; Kp input double; Kd input double
function tau   = computeTorque(DoFs,q,q0,dq,M,h,h0,J,JdotNu,ddx,ddw,epsilon,Kp,Kd)

    Dofs = 11;
    
    Sb = zeros(Dofs,6);
    Ss = eye(Dofs);
    S = [Sb Ss]';

    ddX = [ddx' 0 0 0]';

    %%Primary Task
    lambda = (J(1:3,:)/M)*S;
    alpha = pinvDamped(lambda,epsilon);
    
    tau_pri = alpha*(ddX(1:3) - JdotNu(1:3) + (J(1:3,:)/M)*h);
    
    nullspace = eye(size(lambda,2)) - alpha*lambda;
    
    %%Postural Task
    kp = Kp;
    kd = Kd;
    tau_null = S'*h - kp*(q-q0) - kd*(dq);
    
    tau = tau_pri + nullspace*tau_null;

end

== matlab function Human System/References/Orientation Control Objective/Rotational PID ==
  data: w_R_b_des input double; w_R_b input double; w_omega input double; omegaDot_star output double; Kp input double; Kd input double
function omegaDot_star = rotPID(w_R_b_des,w_R_b,w_omega,Kp,Kd)

    w_omega_des = [0;0;0];
    w_omegaDot_des = [0;0;0];
    
    omegaDot_star = rotationalPID(w_R_b,w_omega,w_R_b_des,w_omega_des,w_omegaDot_des,Kp,Kd);
end

== matlab function Human System/References/Position Control Objective ==
  data: W_H_EE input double; ddx output double; W_J_EE input double; dq input double; x_des input double; dx_des input double; ddx_des input double; Kp input double; Kd input double
function ddx = controlObjective(W_H_EE,W_J_EE,dq,x_des,dx_des,ddx_des,Kp,Kd)
   
    x  = W_H_EE(1:3,4)-x_des;
    dx = W_J_EE(1:3,7:end)*dq-dx_des;
    
    ddx = ddx_des-Kp*x-Kd*dx; 

end

== matlab function Human System/References/Task reference/Real time plot/Position Error Plots  ==
  data: viz_flag input double; sim_time input double; Xactual input double; Xdesired input double
function positionErrorPlots(viz_flag,sim_time,Xactual,Xdesired)
%#codegen

coder.extrinsic('animatedline')
coder.extrinsic('addpoints')
coder.extrinsic('legend')
coder.extrinsic('clearpoints')

if(viz_flag ~= 0)
    
    Xerror = Xactual - Xdesired;
    curve_position_error = animatedline('LineWidth',0.1,'Marker','+');

    if(sim_time == 0)
    
        clf;
        close;
    
        fig1 = figure;
        view(177,15); hold on;
        grid on;
        xlabel('x');
        ylabel('y');
        zlabel('z');
        title('Position Error'); hold on;
% %         axis([-0.3 0.3 -0.3 0.3 -0.3 0.3]);
       
    end
    
    figure(1);
    addpoints(curve_position_error,Xerror(1),Xerror(2),Xerror(3));
    drawnow;
    
end

end

== matlab function comPositeMatrices ==
  data: robotM input double; robotBiasForce input double; humanM input double; humanBiasForce input double; robotEEJ input double; humanEEJ input double; extWrench input double; robotJDotNu input double; humanJDotNu input double
function compositeMatrices(robotM,robotBiasForce,humanM,humanBiasForce,robotEEJ,humanEEJ,extWrench,robotJDotNu,humanJDotNu)

    M = [humanM zeros(17);
         zeros(17) robotM];
     
    h = [humanBiasForce;
         robotBiasForce];
     
    humanB = [zeros(11,6) eye(11)]';
    robotB = [zeros(11,6) eye(11)]';
    
    B = [humanB zeros(17,11);
         zeros(17,11) robotB];
     
    J = [humanEEJ' zeros(17,6);
          zeros(17,6) robotEEJ']';
      
    f = [extWrench; -extWrench];
    
    PV = [robotJDotNu-humanJDotNu];
    
    Q = [humanEEJ-robotEEJ];
    
end
